simulink model "PlanarRobot5link_changedconstraint"  (R2022b)
settings: Solver=VariableStepAuto  StartTime=0.0  StopTime=100  RelTol=1e-3
values from neighbouring files (symbols this model uses):
  I = [1; 1; 1; 0.5; 0.5]*0.2    [RobDyn4link.m]
  l = [1; 1; 1; 1; 2]*0.2    [RobDyn4link.m]
  lc = l./2    [RobDyn4link.m]
  m = [1; 1; 1; 0.3; 0.3]*1    [RobDyn4link.m]
  q0 = [pi/2; -pi/4; -1*pi/6;-pi/12;0;]    [RobDyn4link.m]
  theta_max = [0.915*pi; 0.915*pi; 0.915*pi; 0.915*pi; 0.915*pi;]    [RobDyn4link.m]
  theta_min = [-0.915*pi; -0.915*pi; -0.915*pi; -0.915*pi; -0.915*pi;]    [RobDyn4link.m]
libraries: slpidlib x2
(part 3 of 3)

== matlab function PlanarRobot5link_changedconstraint/Subsystem6/Subsystem/MATLAB Function ==
  data: theta input; M output; l input; lc input; I input; m input; Minv output
function [M,Minv] = fcn(theta,l,lc,I,m)
theta1 = theta(1); theta2 = theta(2); theta3 = theta(3); theta4 = theta(4); theta5 = theta(5);
% dtheta1 = dtheta(1); dtheta2 = dtheta(2); dtheta3 = dtheta(3); dtheta4 = dtheta(4); dtheta5 = dtheta(5);
I1 = I(1); I2 = I(2); I3 = I(3); I4 = I(4); I5 = I(5);
m1 = m(1); m2 = m(2); m3 = m(3); m4 = m(4); m5 = m(5);
l1 = l(1); l2 = l(2); l3 = l(3); l4 = l(4); l5 = l(5);
lc1 = lc(1); lc2 = lc(2); lc3 = lc(3); lc4 = lc(4); lc5 = lc(5);
% M = zeros(5,5);
% M(1,1) = I1 + I2 + I3 + I4 + I5 + l1^2*m2 + l1^2*m3 + l1^2*m4 + l2^2*m3 + l1^2*m5 + l2^2*m4 + l2^2*m5 + l3^2*m4 + l3^2*m5 + l4^2*m5 + lc1^2*m1 + lc2^2*m2 + lc3^2*m3 + lc4^2*m4 + lc5^2*m5 + 2*l1*lc5*m5*cos(theta2 + theta3 + theta4 + theta5) + 2*l1*l3*m4*cos(theta2 + theta3) + 2*l1*l3*m5*cos(theta2 + theta3) + 2*l2*l4*m5*cos(theta3 + theta4) + 2*l1*lc3*m3*cos(theta2 + theta3) + 2*l2*lc4*m4*cos(theta3 + theta4) + 2*l3*lc5*m5*cos(theta4 + theta5) + 2*l1*l2*m3*cos(theta2) + 2*l1*l2*m4*cos(theta2) + 2*l1*l2*m5*cos(theta2) + 2*l2*l3*m4*cos(theta3) + 2*l2*l3*m5*cos(theta3) + 2*l3*l4*m5*cos(theta4) + 2*l1*lc2*m2*cos(theta2) + 2*l2*lc3*m3*cos(theta3) + 2*l3*lc4*m4*cos(theta4) + 2*l4*lc5*m5*cos(theta5) + 2*l1*l4*m5*cos(theta2 + theta3 + theta4) + 2*l1*lc4*m4*cos(theta2 + theta3 + theta4) + 2*l2*lc5*m5*cos(theta3 + theta4 + theta5);
% M(1,2) = I2 + I3 + I4 + I5 + l2^2*m3 + l2^2*m4 + l2^2*m5 + l3^2*m4 + l3^2*m5 + l4^2*m5 + lc2^2*m2 + lc3^2*m3 + lc4^2*m4 + lc5^2*m5 + l1*lc5*m5*cos(theta2 + theta3 + theta4 + theta5) + l1*l3*m4*cos(theta2 + theta3) + l1*l3*m5*cos(theta2 + theta3) + 2*l2*l4*m5*cos(theta3 + theta4) + l1*lc3*m3*cos(theta2 + theta3) + 2*l2*lc4*m4*cos(theta3 + theta4) + 2*l3*lc5*m5*cos(theta4 + theta5) + l1*l2*m3*cos(theta2) + l1*l2*m4*cos(theta2) + l1*l2*m5*cos(theta2) + 2*l2*l3*m4*cos(theta3) + 2*l2*l3*m5*cos(theta3) + 2*l3*l4*m5*cos(theta4) + l1*lc2*m2*cos(theta2) + 2*l2*lc3*m3*cos(theta3) + 2*l3*lc4*m4*cos(theta4) + 2*l4*lc5*m5*cos(theta5) + l1*l4*m5*cos(theta2 + theta3 + theta4) + l1*lc4*m4*cos(theta2 + theta3 + theta4) + 2*l2*lc5*m5*cos(theta3 + theta4 + theta5);
% M(1,3) = I3 + I4 + I5 + l3^2*m4 + l3^2*m5 + l4^2*m5 + lc3^2*m3 + lc4^2*m4 + lc5^2*m5 + l1*lc5*m5*cos(theta2 + theta3 + theta4 + theta5) + l1*l3*m4*cos(theta2 + theta3) + l1*l3*m5*cos(theta2 + theta3) + l2*l4*m5*cos(theta3 + theta4) + l1*lc3*m3*cos(theta2 + theta3) + l2*lc4*m4*cos(theta3 + theta4) + 2*l3*lc5*m5*cos(theta4 + theta5) + l2*l3*m4*cos(theta3) + l2*l3*m5*cos(theta3) + 2*l3*l4*m5*cos(theta4) + l2*lc3*m3*cos(theta3) + 2*l3*lc4*m4*cos(theta4) + 2*l4*lc5*m5*cos(theta5) + l1*l4*m5*cos(theta2 + theta3 + theta4) + l1*lc4*m4*cos(theta2 + theta3 + theta4) + l2*lc5*m5*cos(theta3 + theta4 + theta5);
% M(1,4) = I4 + I5 + l4^2*m5 + lc4^2*m4 + lc5^2*m5 + l1*lc5*m5*cos(theta2 + theta3 + theta4 + theta5) + l2*l4*m5*cos(theta3 + theta4) + l2*lc4*m4*cos(theta3 + theta4) + l3*lc5*m5*cos(theta4 + theta5) + l3*l4*m5*cos(theta4) + l3*lc4*m4*cos(theta4) + 2*l4*lc5*m5*cos(theta5) + l1*l4*m5*cos(theta2 + theta3 + theta4) + l1*lc4*m4*cos(theta2 + theta3 + theta4) + l2*lc5*m5*cos(theta3 + theta4 + theta5);
% M(1,5) = I5 + lc5^2*m5 + l1*lc5*m5*cos(theta2 + theta3 + theta4 + theta5) + l3*lc5*m5*cos(theta4 + theta5) + l4*lc5*m5*cos(theta5) + l2*lc5*m5*cos(theta3 + theta4 + theta5);
% M(2,1) = M(1,1);
% M(2,2) = I2 + I3 + I4 + I5 + l2^2*m3 + l2^2*m4 + l2^2*m5 + l3^2*m4 + l3^2*m5 + l4^2*m5 + lc2^2*m2 + lc3^2*m3 + lc4^2*m4 + lc5^2*m5 + 2*l2*l4*m5*cos(theta3 + theta4) + 2*l2*lc4*m4*cos(theta3 + theta4) + 2*l3*lc5*m5*cos(theta4 + theta5) + 2*l2*l3*m4*cos(theta3) + 2*l2*l3*m5*cos(theta3) + 2*l3*l4*m5*cos(theta4) + 2*l2*lc3*m3*cos(theta3) + 2*l3*lc4*m4*cos(theta4) + 2*l4*lc5*m5*cos(theta5) + 2*l2*lc5*m5*cos(theta3 + theta4 + theta5);
% M(2,3) = I3 + I4 + I5 + l3^2*m4 + l3^2*m5 + l4^2*m5 + lc3^2*m3 + lc4^2*m4 + lc5^2*m5 + l2*l4*m5*cos(theta3 + theta4) + l2*lc4*m4*cos(theta3 + theta4) + 2*l3*lc5*m5*cos(theta4 + theta5) + l2*l3*m4*cos(theta3) + l2*l3*m5*cos(theta3) + 2*l3*l4*m5*cos(theta4) + l2*lc3*m3*cos(theta3) + 2*l3*lc4*m4*cos(theta4) + 2*l4*lc5*m5*cos(theta5) + l2*lc5*m5*cos(theta3 + theta4 + theta5);
% M(2,4) = I4 + I5 + l4^2*m5 + lc4^2*m4 + lc5^2*m5 + l2*l4*m5*cos(theta3 + theta4) + l2*lc4*m4*cos(theta3 + theta4) + l3*lc5*m5*cos(theta4 + theta5) + l3*l4*m5*cos(theta4) + l3*lc4*m4*cos(theta4) + 2*l4*lc5*m5*cos(theta5) + l2*lc5*m5*cos(theta3 + theta4 + theta5);
% M(2,5) = I5 + lc5^2*m5 + l3*lc5*m5*cos(theta4 + theta5) + l4*lc5*m5*cos(theta5) + l2*lc5*m5*cos(theta3 + theta4 + theta5);
% M(3,1) = M(1,3);
% M(3,2) = M(2,3);
% M(3,3) = I3 + I4 + I5 + l3^2*m4 + l3^2*m5 + lc3^2*m3 + lc4^2*m4 + lc4^2*m5 + lc5^2*m5 + 2*l3*lc5*m5*cos(theta4 + theta5) + 2*l3*lc4*m4*cos(theta4) + 2*l3*lc4*m5*cos(theta4) + 2*lc4*lc5*m5*cos(theta5);
% M(3,4) = m5*l4^2 + 2*m5*cos(theta5)*l4*lc5 + l3*m5*cos(theta4)*l4 + m4*lc4^2 + l3*m4*cos(theta4)*lc4 + m5*lc5^2 + l3*m5*cos(theta4 + theta5)*lc5 + I4 + I5;
% M(3,5) = I5 + lc5^2*m5 + l3*lc5*m5*cos(theta4 + theta5) + l4*lc5*m5*cos(theta5);
% M(4,1) = M(1,4);
% M(4,2) = M(2,4);
% M(4,3) = M(3,4);
% M(4,4) = m5*l4^2 + 2*m5*cos(theta5)*l4*lc5 + m4*lc4^2 + m5*lc5^2 + I4 + I5;
% M(4,5) = m5*lc5^2 + l4*m5*cos(theta5)*lc5 + I5;
% M(5,1) = M(1,5);
% M(5,2) = M(2,5);
% M(5,3) = M(3,5);
% M(5,4) = M(4,5);
% M(5,5) = m5*lc5^2 + I5;

M = [I1 + I2 + I3 + I4 + I5 + l1^2*m2 + l1^2*m3 + l1^2*m4 + l2^2*m3 + l1^2*m5 + l2^2*m4 + l2^2*m5 + l3^2*m4 + l3^2*m5 + l4^2*m5 + lc1^2*m1 + lc2^2*m2 + lc3^2*m3 + lc4^2*m4 + lc5^2*m5 + 2*l1*lc5*m5*cos(theta2 + theta3 + theta4 + theta5) + 2*l1*l3*m4*cos(theta2 + theta3) + 2*l1*l3*m5*cos(theta2 + theta3) + 2*l2*l4*m5*cos(theta3 + theta4) + 2*l1*lc3*m3*cos(theta2 + theta3) + 2*l2*lc4*m4*cos(theta3 + theta4) + 2*l3*lc5*m5*cos(theta4 + theta5) + 2*l1*l2*m3*cos(theta2) + 2*l1*l2*m4*cos(theta2) + 2*l1*l2*m5*cos(theta2) + 2*l2*l3*m4*cos(theta3) + 2*l2*l3*m5*cos(theta3) + 2*l3*l4*m5*cos(theta4) + 2*l1*lc2*m2*cos(theta2) + 2*l2*lc3*m3*cos(theta3) + 2*l3*lc4*m4*cos(theta4) + 2*l4*lc5*m5*cos(theta5) + 2*l1*l4*m5*cos(theta2 + theta3 + theta4) + 2*l1*lc4*m4*cos(theta2 + theta3 + theta4) + 2*l2*lc5*m5*cos(theta3 + theta4 + theta5), I2 + I3 + I4 + I5 + l2^2*m3 + l2^2*m4 + l2^2*m5 + l3^2*m4 + l3^2*m5 + l4^2*m5 + lc2^2*m2 + lc3^2*m3 + lc4^2*m4 + lc5^2*m5 + l1*lc5*m5*cos(theta2 + theta3 + theta4 + theta5) + l1*l3*m4*cos(theta2 + theta3) + l1*l3*m5*cos(theta2 + theta3) + 2*l2*l4*m5*cos(theta3 + theta4) + l1*lc3*m3*cos(theta2 + theta3) + 2*l2*lc4*m4*cos(theta3 + theta4) + 2*l3*lc5*m5*cos(theta4 + theta5) + l1*l2*m3*cos(theta2) + l1*l2*m4*cos(theta2) + l1*l2*m5*cos(theta2) + 2*l2*l3*m4*cos(theta3) + 2*l2*l3*m5*cos(theta3) + 2*l3*l4*m5*cos(theta4) + l1*lc2*m2*cos(theta2) + 2*l2*lc3*m3*cos(theta3) + 2*l3*lc4*m4*cos(theta4) + 2*l4*lc5*m5*cos(theta5) + l1*l4*m5*cos(theta2 + theta3 + theta4) + l1*lc4*m4*cos(theta2 + theta3 + theta4) + 2*l2*lc5*m5*cos(theta3 + theta4 + theta5), I3 + I4 + I5 + l3^2*m4 + l3^2*m5 + l4^2*m5 + lc3^2*m3 + lc4^2*m4 + lc5^2*m5 + l1*lc5*m5*cos(theta2 + theta3 + theta4 + theta5) + l1*l3*m4*cos(theta2 + theta3) + l1*l3*m5*cos(theta2 + theta3) + l2*l4*m5*cos(theta3 + theta4) + l1*lc3*m3*cos(theta2 + theta3) + l2*lc4*m4*cos(theta3 + theta4) + 2*l3*lc5*m5*cos(theta4 + theta5) + l2*l3*m4*cos(theta3) + l2*l3*m5*cos(theta3) + 2*l3*l4*m5*cos(theta4) + l2*lc3*m3*cos(theta3) + 2*l3*lc4*m4*cos(theta4) + 2*l4*lc5*m5*cos(theta5) + l1*l4*m5*cos(theta2 + theta3 + theta4) + l1*lc4*m4*cos(theta2 + theta3 + theta4) + l2*lc5*m5*cos(theta3 + theta4 + theta5), I4 + I5 + l4^2*m5 + lc4^2*m4 + lc5^2*m5 + l1*lc5*m5*cos(theta2 + theta3 + theta4 + theta5) + l2*l4*m5*cos(theta3 + theta4) + l2*lc4*m4*cos(theta3 + theta4) + l3*lc5*m5*cos(theta4 + theta5) + l3*l4*m5*cos(theta4) + l3*lc4*m4*cos(theta4) + 2*l4*lc5*m5*cos(theta5) + l1*l4*m5*cos(theta2 + theta3 + theta4) + l1*lc4*m4*cos(theta2 + theta3 + theta4) + l2*lc5*m5*cos(theta3 + theta4 + theta5), I5 + lc5^2*m5 + l1*lc5*m5*cos(theta2 + theta3 + theta4 + theta5) + l3*lc5*m5*cos(theta4 + theta5) + l4*lc5*m5*cos(theta5) + l2*lc5*m5*cos(theta3 + theta4 + theta5);
                                                                            I2 + I3 + I4 + I5 + l2^2*m3 + l2^2*m4 + l2^2*m5 + l3^2*m4 + l3^2*m5 + l4^2*m5 + lc2^2*m2 + lc3^2*m3 + lc4^2*m4 + lc5^2*m5 + l1*lc5*m5*cos(theta2 + theta3 + theta4 + theta5) + l1*l3*m4*cos(theta2 + theta3) + l1*l3*m5*cos(theta2 + theta3) + 2*l2*l4*m5*cos(theta3 + theta4) + l1*lc3*m3*cos(theta2 + theta3) + 2*l2*lc4*m4*cos(theta3 + theta4) + 2*l3*lc5*m5*cos(theta4 + theta5) + l1*l2*m3*cos(theta2) + l1*l2*m4*cos(theta2) + l1*l2*m5*cos(theta2) + 2*l2*l3*m4*cos(theta3) + 2*l2*l3*m5*cos(theta3) + 2*l3*l4*m5*cos(theta4) + l1*lc2*m2*cos(theta2) + 2*l2*lc3*m3*cos(theta3) + 2*l3*lc4*m4*cos(theta4) + 2*l4*lc5*m5*cos(theta5) + l1*l4*m5*cos(theta2 + theta3 + theta4) + l1*lc4*m4*cos(theta2 + theta3 + theta4) + 2*l2*lc5*m5*cos(theta3 + theta4 + theta5),                                                                                                                                                                                                                                                                                                                                     I2 + I3 + I4 + I5 + l2^2*m3 + l2^2*m4 + l2^2*m5 + l3^2*m4 + l3^2*m5 + l4^2*m5 + lc2^2*m2 + lc3^2*m3 + lc4^2*m4 + lc5^2*m5 + 2*l2*l4*m5*cos(theta3 + theta4) + 2*l2*lc4*m4*cos(theta3 + theta4) + 2*l3*lc5*m5*cos(theta4 + theta5) + 2*l2*l3*m4*cos(theta3) + 2*l2*l3*m5*cos(theta3) + 2*l3*l4*m5*cos(theta4) + 2*l2*lc3*m3*cos(theta3) + 2*l3*lc4*m4*cos(theta4) + 2*l4*lc5*m5*cos(theta5) + 2*l2*lc5*m5*cos(theta3 + theta4 + theta5),                                                                                                                                                                                                                                        I3 + I4 + I5 + l3^2*m4 + l3^2*m5 + l4^2*m5 + lc3^2*m3 + lc4^2*m4 + lc5^2*m5 + l2*l4*m5*cos(theta3 + theta4) + l2*lc4*m4*cos(theta3 + theta4) + 2*l3*lc5*m5*cos(theta4 + theta5) + l2*l3*m4*cos(theta3) + l2*l3*m5*cos(theta3) + 2*l3*l4*m5*cos(theta4) + l2*lc3*m3*cos(theta3) + 2*l3*lc4*m4*cos(theta4) + 2*l4*lc5*m5*cos(theta5) + l2*lc5*m5*cos(theta3 + theta4 + theta5),                                                                                                                                       I4 + I5 + l4^2*m5 + lc4^2*m4 + lc5^2*m5 + l2*l4*m5*cos(theta3 + theta4) + l2*lc4*m4*cos(theta3 + theta4) + l3*lc5*m5*cos(theta4 + theta5) + l3*l4*m5*cos(theta4) + l3*lc4*m4*cos(theta4) + 2*l4*lc5*m5*cos(theta5) + l2*lc5*m5*cos(theta3 + theta4 + theta5),                                                    I5 + lc5^2*m5 + l3*lc5*m5*cos(theta4 + theta5) + l4*lc5*m5*cos(theta5) + l2*lc5*m5*cos(theta3 + theta4 + theta5);
                                                                                                                                                                                                                                   I3 + I4 + I5 + l3^2*m4 + l3^2*m5 + l4^2*m5 + lc3^2*m3 + lc4^2*m4 + lc5^2*m5 + l1*lc5*m5*cos(theta2 + theta3 + theta4 + theta5) + l1*l3*m4*cos(theta2 + theta3) + l1*l3*m5*cos(theta2 + theta3) + l2*l4*m5*cos(theta3 + theta4) + l1*lc3*m3*cos(theta2 + theta3) + l2*lc4*m4*cos(theta3 + theta4) + 2*l3*lc5*m5*cos(theta4 + theta5) + l2*l3*m4*cos(theta3) + l2*l3*m5*cos(theta3) + 2*l3*l4*m5*cos(theta4) + l2*lc3*m3*cos(theta3) + 2*l3*lc4*m4*cos(theta4) + 2*l4*lc5*m5*cos(theta5) + l1*l4*m5*cos(theta2 + theta3 + theta4) + l1*lc4*m4*cos(theta2 + theta3 + theta4) + l2*lc5*m5*cos(theta3 + theta4 + theta5),                                                                                                                                                                                                                                                                                                                                                                                               I3 + I4 + I5 + l3^2*m4 + l3^2*m5 + l4^2*m5 + lc3^2*m3 + lc4^2*m4 + lc5^2*m5 + l2*l4*m5*cos(theta3 + theta4) + l2*lc4*m4*cos(theta3 + theta4) + 2*l3*lc5*m5*cos(theta4 + theta5) + l2*l3*m4*cos(theta3) + l2*l3*m5*cos(theta3) + 2*l3*l4*m5*cos(theta4) + l2*lc3*m3*cos(theta3) + 2*l3*lc4*m4*cos(theta4) + 2*l4*lc5*m5*cos(theta5) + l2*lc5*m5*cos(theta3 + theta4 + theta5),                                                                                                                                                                                                                                                                                                                                                                                                                         I3 + I4 + I5 + l3^2*m4 + l3^2*m5 + l4^2*m5 + lc3^2*m3 + lc4^2*m4 + lc5^2*m5 + 2*l3*lc5*m5*cos(theta4 + theta5) + 2*l3*l4*m5*cos(theta4) + 2*l3*lc4*m4*cos(theta4) + 2*l4*lc5*m5*cos(theta5),                                                                                                                                                                                                                                                  m5*l4^2 + 2*m5*cos(theta5)*l4*lc5 + l3*m5*cos(theta4)*l4 + m4*lc4^2 + l3*m4*cos(theta4)*lc4 + m5*lc5^2 + l3*m5*cos(theta4 + theta5)*lc5 + I4 + I5,                                                                                              I5 + lc5^2*m5 + l3*lc5*m5*cos(theta4 + theta5) + l4*lc5*m5*cos(theta5);
                                                                                                                                                                                                                                                                                                                                                                                                                                                    I4 + I5 + l4^2*m5 + lc4^2*m4 + lc5^2*m5 + l1*lc5*m5*cos(theta2 + theta3 + theta4 + theta5) + l2*l4*m5*cos(theta3 + theta4) + l2*lc4*m4*cos(theta3 + theta4) + l3*lc5*m5*cos(theta4 + theta5) + l3*l4*m5*cos(theta4) + l3*lc4*m4*cos(theta4) + 2*l4*lc5*m5*cos(theta5) + l1*l4*m5*cos(theta2 + theta3 + theta4) + l1*lc4*m4*cos(theta2 + theta3 + theta4) + l2*lc5*m5*cos(theta3 + theta4 + theta5),                                                                                                                                                                                                                                                                                                                                                                                                                                                                                                               I4 + I5 + l4^2*m5 + lc4^2*m4 + lc5^2*m5 + l2*l4*m5*cos(theta3 + theta4) + l2*lc4*m4*cos(theta3 + theta4) + l3*lc5*m5*cos(theta4 + theta5) + l3*l4*m5*cos(theta4) + l3*lc4*m4*cos(theta4) + 2*l4*lc5*m5*cos(theta5) + l2*lc5*m5*cos(theta3 + theta4 + theta5),                                                                                                                                                                                                                                                                                                                                                                                                                                                                   m5*l4^2 + 2*m5*cos(theta5)*l4*lc5 + l3*m5*cos(theta4)*l4 + m4*lc4^2 + l3*m4*cos(theta4)*lc4 + m5*lc5^2 + l3*m5*cos(theta4 + theta5)*lc5 + I4 + I5,                                                                                                                                                                                                                                                                                                                                  m5*l4^2 + 2*m5*cos(theta5)*l4*lc5 + m4*lc4^2 + m5*lc5^2 + I4 + I5,                                                                                                                               m5*lc5^2 + l4*m5*cos(theta5)*lc5 + I5;
                                                                                                                                                                                                                                                                                                                                                                                                                                                                                                                                                                                                                                                                                   I5 + lc5^2*m5 + l1*lc5*m5*cos(theta2 + theta3 + theta4 + theta5) + l3*lc5*m5*cos(theta4 + theta5) + l4*lc5*m5*cos(theta5) + l2*lc5*m5*cos(theta3 + theta4 + theta5),                                                                                                                                                                                                                                                                                                                                                                                                                                                                                                                                                                                                                                                           I5 + lc5^2*m5 + l3*lc5*m5*cos(theta4 + theta5) + l4*lc5*m5*cos(theta5) + l2*lc5*m5*cos(theta3 + theta4 + theta5),                                                                                                                                                                                                                                                                                                                                                                                                                                                                                                                                              I5 + lc5^2*m5 + l3*lc5*m5*cos(theta4 + theta5) + l4*lc5*m5*cos(theta5),                                                                                                                                                                                                                                                                                                                                                              m5*lc5^2 + l4*m5*cos(theta5)*lc5 + I5,                                                                                                                                                       m5*lc5^2 + I5;];

Minv = inv(M);

== matlab function PlanarRobot5link_changedconstraint/Subsystem6/Subsystem2/MATLAB Function ==
  data: theta input; G output; m input; l input; lc input
function G = fcn(theta,m,l,lc)
theta1 = theta(1); theta2 = theta(2); theta3 = theta(3); theta4 = theta(4); theta5 = theta(5);
% dtheta1 = dtheta(1); dtheta2 = dtheta(2); dtheta3 = dtheta(3); dtheta4 = dtheta(4); dtheta5 = dtheta(5);
% I1 = I(1); I2 = I(2); I3 = I(3); I4 = I(4); I5 = I(5);
m1 = m(1); m2 = m(2); m3 = m(3); m4 = m(4); m5 = m(5);
l1 = l(1); l2 = l(2); l3 = l(3); l4 = l(4); l5 = l(5);
lc1 = lc(1); lc2 = lc(2); lc3 = lc(3); lc4 = lc(4); lc5 = lc(5);
g = 9.81;

G = [g*l4*m4*cos(theta1 + theta2 + theta3 + theta4) + g*lc4*m4*cos(theta1 + theta2 + theta3 + theta4) + g*l2*m3*cos(theta1 + theta2) + 2*g*l2*m4*cos(theta1 + theta2) + g*lc2*m2*cos(theta1 + theta2) + g*l1*m2*cos(theta1) + g*l1*m3*cos(theta1) + 2*g*l1*m4*cos(theta1) + g*lc1*m1*cos(theta1) + g*lc5*m4*cos(theta1 + theta2 + theta3 + theta4 + theta5) + 2*g*l3*m4*cos(theta1 + theta2 + theta3) + g*lc3*m3*cos(theta1 + theta2 + theta3);
                                                                                           g*l4*m4*cos(theta1 + theta2 + theta3 + theta4) + g*lc4*m4*cos(theta1 + theta2 + theta3 + theta4) + g*l2*m3*cos(theta1 + theta2) + 2*g*l2*m4*cos(theta1 + theta2) + g*lc2*m2*cos(theta1 + theta2) + g*lc5*m4*cos(theta1 + theta2 + theta3 + theta4 + theta5) + 2*g*l3*m4*cos(theta1 + theta2 + theta3) + g*lc3*m3*cos(theta1 + theta2 + theta3);
                                                                                                                                                                                           g*l4*m4*cos(theta1 + theta2 + theta3 + theta4) + g*lc4*m4*cos(theta1 + theta2 + theta3 + theta4) + g*lc5*m4*cos(theta1 + theta2 + theta3 + theta4 + theta5) + 2*g*l3*m4*cos(theta1 + theta2 + theta3) + g*lc3*m3*cos(theta1 + theta2 + theta3);
                                                                                                                                                                                                                                                                                 g*m4*(l4*cos(theta1 + theta2 + theta3 + theta4) + lc5*cos(theta1 + theta2 + theta3 + theta4 + theta5)) + g*lc4*m4*cos(theta1 + theta2 + theta3 + theta4);
                                                                                                                                                                                                                                                                                                                                                                                 g*lc5*m4*cos(theta1 + theta2 + theta3 + theta4 + theta5)];

== matlab function PlanarRobot5link_changedconstraint/Subsystem6/Subsystem4/MATLAB Function ==
  data: theta input; J5e output; l input; J5 output; J4e output; J4 output
function [J5e,J5,J4e,J4] = fcn(theta,l)
l1 = l(1); l2 = l(2); l3 = l(3); l4 = l(4); l5 = l(5);
theta1 = theta(1); theta2 = theta(2); theta3 = theta(3); theta4 = theta(4); theta5 = theta(5);



J5e = [- l4*sin(theta1 + theta2 + theta3 + theta4) - l2*sin(theta1 + theta2) - l1*sin(theta1) - l5*sin(theta1 + theta2 + theta3 + theta4 + theta5) - l3*sin(theta1 + theta2 + theta3), - l4*sin(theta1 + theta2 + theta3 + theta4) - l2*sin(theta1 + theta2) - l5*sin(theta1 + theta2 + theta3 + theta4 + theta5) - l3*sin(theta1 + theta2 + theta3), - l4*sin(theta1 + theta2 + theta3 + theta4) - l5*sin(theta1 + theta2 + theta3 + theta4 + theta5) - l3*sin(theta1 + theta2 + theta3), - l4*sin(theta1 + theta2 + theta3 + theta4) - l5*sin(theta1 + theta2 + theta3 + theta4 + theta5), -l5*sin(theta1 + theta2 + theta3 + theta4 + theta5);
  l4*cos(theta1 + theta2 + theta3 + theta4) + l2*cos(theta1 + theta2) + l1*cos(theta1) + l5*cos(theta1 + theta2 + theta3 + theta4 + theta5) + l3*cos(theta1 + theta2 + theta3),   l4*cos(theta1 + theta2 + theta3 + theta4) + l2*cos(theta1 + theta2) + l5*cos(theta1 + theta2 + theta3 + theta4 + theta5) + l3*cos(theta1 + theta2 + theta3),   l4*cos(theta1 + theta2 + theta3 + theta4) + l5*cos(theta1 + theta2 + theta3 + theta4 + theta5) + l3*cos(theta1 + theta2 + theta3),   l4*cos(theta1 + theta2 + theta3 + theta4) + l5*cos(theta1 + theta2 + theta3 + theta4 + theta5),  l5*cos(theta1 + theta2 + theta3 + theta4 + theta5);
                                                                                                                                                                             1,                                                                                                                                                             1,                                                                                                                                   1,                                                                                                1,                                                   1;];
J5 =  [- l4*sin(theta1 + theta2 + theta3 + theta4) - l2*sin(theta1 + theta2) - l1*sin(theta1) - l3*sin(theta1 + theta2 + theta3), - l4*sin(theta1 + theta2 + theta3 + theta4) - l2*sin(theta1 + theta2) - l3*sin(theta1 + theta2 + theta3), - l4*sin(theta1 + theta2 + theta3 + theta4) - l3*sin(theta1 + theta2 + theta3), -l4*sin(theta1 + theta2 + theta3 + theta4), 0;
  l4*cos(theta1 + theta2 + theta3 + theta4) + l2*cos(theta1 + theta2) + l1*cos(theta1) + l3*cos(theta1 + theta2 + theta3),   l4*cos(theta1 + theta2 + theta3 + theta4) + l2*cos(theta1 + theta2) + l3*cos(theta1 + theta2 + theta3),   l4*cos(theta1 + theta2 + theta3 + theta4) + l3*cos(theta1 + theta2 + theta3),  l4*cos(theta1 + theta2 + theta3 + theta4), 0;
                                                                                                                        1,                                                                                                        1,                                                                              1,                                          1, 1];
J4e = [- l4*sin(theta1 + theta2 + theta3 + theta4) - l2*sin(theta1 + theta2) - l1*sin(theta1) - l3*sin(theta1 + theta2 + theta3), - l4*sin(theta1 + theta2 + theta3 + theta4) - l2*sin(theta1 + theta2) - l3*sin(theta1 + theta2 + theta3), - l4*sin(theta1 + theta2 + theta3 + theta4) - l3*sin(theta1 + theta2 + theta3), -l4*sin(theta1 + theta2 + theta3 + theta4), 0;
  l4*cos(theta1 + theta2 + theta3 + theta4) + l2*cos(theta1 + theta2) + l1*cos(theta1) + l3*cos(theta1 + theta2 + theta3),   l4*cos(theta1 + theta2 + theta3 + theta4) + l2*cos(theta1 + theta2) + l3*cos(theta1 + theta2 + theta3),   l4*cos(theta1 + theta2 + theta3 + theta4) + l3*cos(theta1 + theta2 + theta3),  l4*cos(theta1 + theta2 + theta3 + theta4), 0;
                                                                                                                        1,                                                                                                        1,                                                                              1,                                          1, 0];
J4 = [- l2*sin(theta1 + theta2) - l1*sin(theta1) - l3*sin(theta1 + theta2 + theta3), - l2*sin(theta1 + theta2) - l3*sin(theta1 + theta2 + theta3), -l3*sin(theta1 + theta2 + theta3), 0, 0;
  l2*cos(theta1 + theta2) + l1*cos(theta1) + l3*cos(theta1 + theta2 + theta3),   l2*cos(theta1 + theta2) + l3*cos(theta1 + theta2 + theta3),  l3*cos(theta1 + theta2 + theta3), 0, 0;
                                                                            1,                                                            1,                                 1, 1, 0];

== matlab function PlanarRobot5link_changedconstraint/Subsystem6/Subsystem5/MATLAB Function ==
  data: x input; y input
function plotManipulator(x, y)
coder.extrinsic('plot5link');
plot5link(x, y)
end

== matlab function PlanarRobot5link_changedconstraint/Subsystem6/Subsystem5/MATLAB Function1 ==
  data: x output; theta input; y output; l input
function [x,y] = fcn(theta,l)
theta1 = theta(1); theta2 = theta(2); theta3 = theta(3); theta4 = theta(4); theta5 = theta(5);
% dtheta1 = dtheta(1); dtheta2 = dtheta(2); dtheta3 = dtheta(3); dtheta4 = dtheta(4); dtheta5 = dtheta(5);
% I1 = I(1); I2 = I(2); I3 = I(3); I4 = I(4); I5 = I(5);
% m1 = m(1); m2 = m(2); m3 = m(3); m4 = m(4); m5 = m(5);
l1 = l(1); l2 = l(2); l3 = l(3); l4 = l(4); l5 = l(5);
% lc1 = lc(1); lc2 = lc(2); lc3 = lc(3); lc4 = lc(4); lc5 = lc(5);

x1 = l1 * cos(theta1);
y1 = l1 * sin(theta1);

x2 = l1 * cos(theta1) + l2 * cos(theta1 + theta2);
y2 = l1 * sin(theta1) + l2 * sin(theta1 + theta2);

x3 = l1 * cos(theta1) + l2 * cos(theta1 + theta2) + l3 * cos(theta1 + theta2 + theta3);
y3 = l1 * sin(theta1) + l2 * sin(theta1 + theta2) + l3 * sin(theta1 + theta2 + theta3);

x4 = l1 * cos(theta1) + l2 * cos(theta1 + theta2) + l3 * cos(theta1 + theta2 + theta3) + l4 * cos(theta1 + theta2 + theta3 + theta4);
y4 = l1 * sin(theta1) + l2 * sin(theta1 + theta2) + l3 * sin(theta1 + theta2 + theta3) + l4 * sin(theta1 + theta2 + theta3 + theta4);

x5 = l1 * cos(theta1) + l2 * cos(theta1 + theta2) + l3 * cos(theta1 + theta2 + theta3) + l4 * cos(theta1 + theta2 + theta3 + theta4) + l5 * cos(theta1 + theta2 + theta3 + theta4 + theta5);
y5 = l1 * sin(theta1) + l2 * sin(theta1 + theta2) + l3 * sin(theta1 + theta2 + theta3) + l4 * sin(theta1 + theta2 + theta3 + theta4) + l5 * sin(theta1 + theta2 + theta3 + theta4 + theta5);

% x6 = l1 * cos(theta1) + l2 * cos(theta1 + theta2) + l3 * cos(theta1 + theta2 + theta3) + l4 * cos(theta1 + theta2 + theta3 + theta4) + l5 * cos(theta1 + theta2 + theta3 + theta4 + theta5);
% y6 = l1 * sin(theta1) + l2 * sin(theta1 + theta2) + l3 * sin(theta1 + theta2 + theta3) + l4 * sin(theta1 + theta2 + theta3 + theta4) + l5 * sin(theta1 + theta2 + theta3 + theta4 + theta5);


x = [0;x1;x2;x3;x4;x5];
y = [0;y1;y2;y3;y4;y5];

== matlab function PlanarRobot5link_changedconstraint/Subsystem/MATLAB Function ==
  data: X_2e_error output; J_2ec output; l input; theta input; J_2eT output; X5e output; X5 output; X4e output
function [X_2e_error,J_2ec,J_2eT,X5e,X5,X4e]= fcn(l,theta)
l1 = l(1); l2 = l(2); l3 = l(3); l4 = l(4); l5 = l(5);
theta1 = theta(1); theta2 = theta(2); theta3 = theta(3); theta4 = theta(4); theta5 = theta(5);

x_2e = l2*cos(theta1 + theta2) + l1*cos(theta1);
y_2e = l2*sin(theta1 + theta2) + l1*sin(theta1);

x_2ed = 0.141421;
y_2ed = 0.341421;

J_2e = [- l2*sin(theta1 + theta2) - l1*sin(theta1), -l2*sin(theta1 + theta2), 0, 0, 0;
  l2*cos(theta1 + theta2) + l1*cos(theta1),  l2*cos(theta1 + theta2), 0, 0, 0;
                                         1,                        1, 0, 0, 0];
J_2ec = J_2e(1:2,:);
X_2e_error = [x_2ed - x_2e; y_2ed - y_2e];
J_2eT = J_2e(1:2,:)';



x5e = l4*cos(theta1 + theta2 + theta3 + theta4) + l2*cos(theta1 + theta2) + l1*cos(theta1) + l5*cos(theta1 + theta2 + theta3 + theta4 + theta5) + l3*cos(theta1 + theta2 + theta3);
y5e = l4*sin(theta1 + theta2 + theta3 + theta4) + l2*sin(theta1 + theta2) + l1*sin(theta1) + l5*sin(theta1 + theta2 + theta3 + theta4 + theta5) + l3*sin(theta1 + theta2 + theta3);
X5e = [x5e;y5e;theta1 + theta2 + theta3 + theta4 + theta5];

x5 = l4*cos(theta1 + theta2 + theta3 + theta4) + l2*cos(theta1 + theta2) + l1*cos(theta1) + l3*cos(theta1 + theta2 + theta3);
y5 = l4*sin(theta1 + theta2 + theta3 + theta4) + l2*sin(theta1 + theta2) + l1*sin(theta1) + l3*sin(theta1 + theta2 + theta3);
X5 = [x5;y5;theta1 + theta2 + theta3 + theta4 + theta5];

x4e = l1 * cos(theta1) + l2 * cos(theta1 + theta2) + l3 * cos(theta1 + theta2 + theta3) + l4 * cos(theta1 + theta2 + theta3 + theta4);
y4e = l1 * sin(theta1) + l2 * sin(theta1 + theta2) + l3 * sin(theta1 + theta2 + theta3) + l4 * sin(theta1 + theta2 + theta3 + theta4);
X4e = [x4e;y4e;theta1 + theta2 + theta3 + theta4];

== matlab function PlanarRobot5link_changedconstraint/Subsystem6/Subsystem3/MATLAB Function ==
  data: theta input; y output; theta_max input; theta_min input
function y = fcn(theta, theta_max, theta_min)
y= max(theta_min,min(theta, theta_max));
